simulink model "showdemuxDims"  (R2024a)
settings: Solver=VariableStepAuto  StartTime=0.0  StopTime=10.0  RelTol=1e-3
settings Model: Creator=grouleau  LastModifiedBy=grouleau

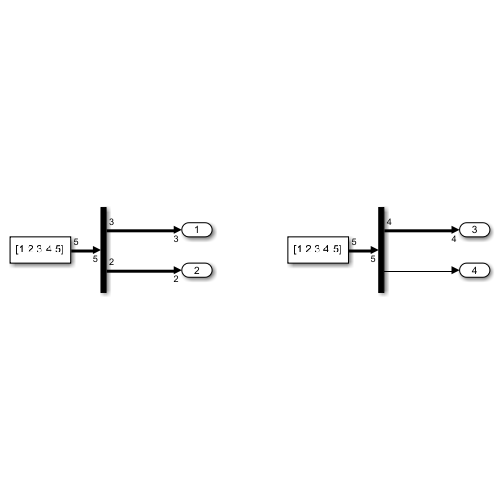
[thumbnail: Simulink's stored preview of the top-level diagram]
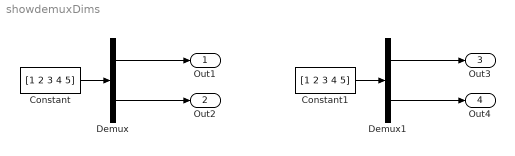
== system showdemuxDims ==
  Constant : Constant  Value=[1 2 3 4 5]
  Constant1 : Constant  Value=[1 2 3 4 5]
  Demux : Demux  Outputs=2
  Demux1 : Demux  Outputs=[4 1]
  Out1 : Outport
  Out2 : Outport  Port=2
  Out3 : Outport  Port=3
  Out4 : Outport  Port=4
  wires:
  Constant/1 -> Demux/1
  Demux/1 -> Out1/1
  Demux/2 -> Out2/1
  Demux1/2 -> Out4/1
  Demux1/1 -> Out3/1
  Constant1/1 -> Demux1/1
